simulink model "inputs"  (R2020a)
settings: Solver=VariableStepAuto  StartTime=0.0  StopTime=10.0  RelTol=1e-3
settings Model: Creator=iwill  LastModifiedBy=iwill

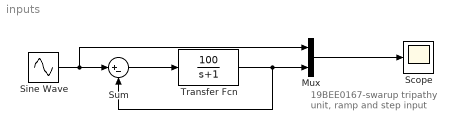
== system inputs ==
  note: 19BEE0167-swarup tripathy
      |
      | unit, ramp and step input
  Mux : Mux  Inputs=2
  Scope : Scope
  Sine Wave : Sin  Frequency=50  SampleTime=0
  Sum : Sum  Inputs=|+-
  Transfer Fcn : TransferFcn  Numerator=[100]  Denominator=[1 1]
  wires:
  Sine Wave/1 -> Mux/1, Sum/1
  Sum/1 -> Transfer Fcn/1
  Transfer Fcn/1 -> Sum/2, Mux/2
  Mux/1 -> Scope/1
